simulink library "Room_Radiator"  (R2013b)
settings: Solver=ode45  StartTime=0.0  StopTime=10.0  RelTol=1e-3
libraries: carnot x17
settings Model: Creator=lena.frank  LastModifiedBy=drhf

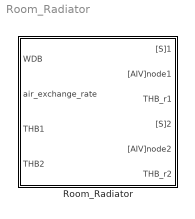
== system Room_Radiator ==
  Room_Radiator : Subsystem  mask(room){t0=20, temp_neighbour=20}
      mask prompts: t0 "start temperature of rooms in °C"; temp_neighbour "temperature of rooms above and below in °C"
      mask help:
      | The block models of a heat transfer characteristic of two neighbour rooms.
      | Use "look under mask" to set up the models parameters (initial conditions,
      | floors and wall characteristics...)
      mask init:
      | AIV_neighbour = [0 temp_neighbour temp_neighbour 0 0 0 0 0 0];
      | zonefloordist2grnd = 0;
      mask Help: web(fullfile(path_carnot('help'),'Room_Radiator.html'),'-helpbrowser')
      mask Display: plot(0,0,100,100,[30,30,60,60,30],[20,50,50,20,20],[47,47,56,56,47],[40,30,30,40,40],[42,42,34,34],[20,40,40,20],[62,45,28],[48,70,48])

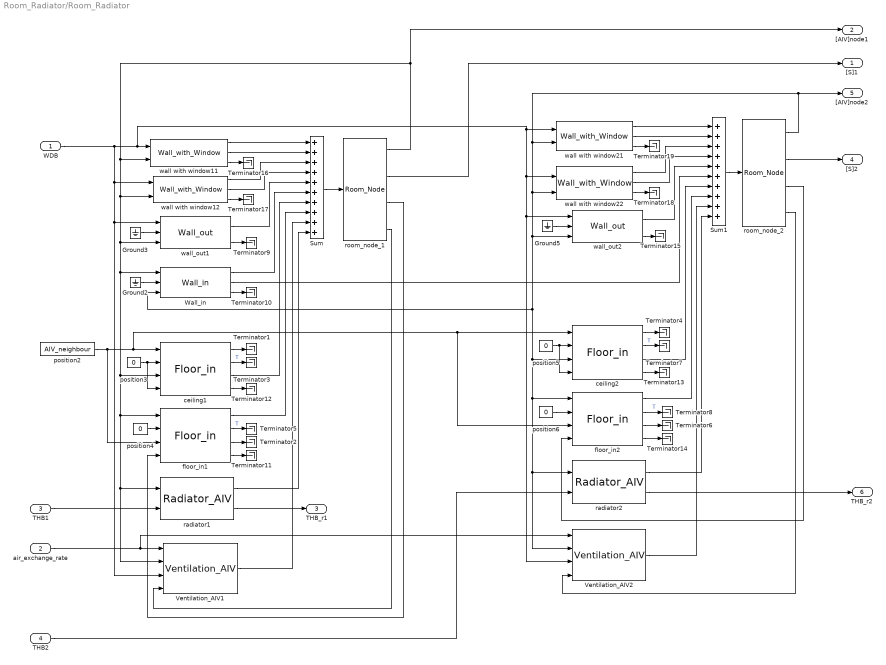
== system Room_Radiator/Room_Radiator ==
  WDB : Inport
  air_exchange_rate : Inport  Port=2
  THB1 : Inport  Port=3
  THB2 : Inport  Port=4
  Ground2 : Ground
  Ground3 : Ground
  Ground5 : Ground
  Sum : Sum  Inputs=10  SaturateOnIntegerOverflow=on  InputSameDT=on  OutDataTypeStr=Inherit: Same as first input
  Sum1 : Sum  Inputs=10  SaturateOnIntegerOverflow=on  InputSameDT=on  OutDataTypeStr=Inherit: Same as first input
  Terminator{1..19} (19 alike) : Terminator
  Ventilation_AIV1 : carnot/Source/Ventilation/Ventilation_AIV  co2=400
  Ventilation_AIV2 : carnot/Source/Ventilation/Ventilation_AIV  co2=400
  Wall_in : carnot/Load/Houses/wall_floor/Wall_in  wallsize=[2.5 5]  d=[0.015 0.38 0.02]  cond=[1.4 0.79 0.7]  cwall=[0.28 0.28 0.28]*3600  rho=[2000 1800 1400]  emission_in=0.96  dactive=-1  t0=20  tau=1000*3600
  ceiling1 : carnot/Load/Houses/wall_floor/Floor_in  wallsize=[5 5]  t0=20  d=[0.015 0.38 0.02]  cond=[1.4 0.79 0.7]  cwall=[0.28 0.28 0.28]*3600  rho=[2000 1800 1400]  misc=[.65 .65]  dactive=-1  tau=1000*3600
  ceiling2 : carnot/Load/Houses/wall_floor/Floor_in  wallsize=[5 5]  t0=20  d=[0.015 0.38 0.02]  cond=[1.4 0.79 0.7]  cwall=[0.28 0.28 0.28]*3600  rho=[2000 1800 1400]  misc=[.65 .65]  dactive=-1  tau=1000*3600
  floor_in1 : carnot/Load/Houses/wall_floor/Floor_in  wallsize=[5 5]  t0=20  d=[0.015 0.38 0.02]  cond=[1.4 0.79 0.7]  cwall=[0.28 0.28 0.28]*3600  rho=[2000 1800 1400]  misc=[.65 .65]  dactive=-1  tau=1000*3600
  floor_in2 : carnot/Load/Houses/wall_floor/Floor_in  wallsize=[5 5]  t0=20  d=[0.015 0.38 0.02]  cond=[1.4 0.79 0.7]  cwall=[0.28 0.28 0.28]*3600  rho=[2000 1800 1400]  misc=[.65 .65]  dactive=-1  tau=1000*3600
  position2 : Constant  Value=AIV_neighbour
  position{3..6} (4 alike) : Constant  Value=0
  radiator1 : carnot/Source/Heat_Exchanger/Radiator_AIV  pnom=500  dtnom=40  expo=1.3  mcap=5*4182  ra=0.47  tini=20  lin=0  qua=1000
  radiator2 : carnot/Source/Heat_Exchanger/Radiator_AIV  pnom=500  dtnom=40  expo=1.3  mcap=5*4182  ra=0.47  tini=20  lin=0  qua=1000
  room_node_1 : carnot/Load/Houses/room_nodes/Room_Node  zoneairvolume=5*5*2.5  zoneheight=2.5  zonestartTEMP=20  zonestartWATER=55  timeconst=100  heatperfect=natural  lookuptime=[0 24]*3600  lookupvalue=[20 20]  AirPressure=101300
  room_node_2 : carnot/Load/Houses/room_nodes/Room_Node  zoneairvolume=5*5*2.5  zoneheight=2.5  zonestartTEMP=20  zonestartWATER=55  timeconst=100  heatperfect=natural  lookuptime=[0 24]*3600  lookupvalue=[20 20]  AirPressure=101300
  wall with window11 : carnot/Load/Houses/wall_floor/Wall_with_Window  wallsize=[2.5 5]  windowsize=[1 2]  frame=0.1  pos=90  t0=20  tau=1000*3600  g=0.7
  wall with window12 : carnot/Load/Houses/wall_floor/Wall_with_Window  wallsize=[2.5 5]  windowsize=[1 2]  frame=0.1  pos=0  t0=20  tau=1000*3600  g=0.7
  wall with window21 : carnot/Load/Houses/wall_floor/Wall_with_Window  wallsize=[2.5 5]  windowsize=[1 2]  frame=0.1  pos=-90  t0=20  tau=1000*3600  g=0.7
  wall with window22 : carnot/Load/Houses/wall_floor/Wall_with_Window  wallsize=[2.5 5]  windowsize=[1 2]  frame=0.1  pos=0  t0=20  tau=1000*3600  g=0.7
  wall_out1 : carnot/Load/Houses/wall_floor/Wall_out  wallsize=[2.5 5]  pos=180  t0=20  d=[0.1 0.38]  cond=[0.04 0.79]  cwall=[0.28 0.28]*3600  rho=[900 1800]  reflectground=0.2  abs_emiss=[0.65 0.97 0.96]  tau=1000*3600  dactive=-1
  wall_out2 : carnot/Load/Houses/wall_floor/Wall_out  wallsize=[2.5 5]  pos=180  t0=20  d=[0.1 0.38]  cond=[0.04 0.79]  cwall=[0.28 0.28]*3600  rho=[900 1800]  reflectground=0.2  abs_emiss=[0.65 0.97 0.96]  tau=1000*3600  dactive=-1
  "[S]1" : Outport
  "[AIV]node1" : Outport  Port=2
  THB_r1 : Outport  Port=3
  "[S]2" : Outport  Port=4
  "[AIV]node2" : Outport  Port=5
  THB_r2 : Outport  Port=6
  wires:
  wall with window21/3 -> Terminator19/1
  wall with window22/3 -> Terminator18/1
  wall with window12/3 -> Terminator17/1
  wall with window11/3 -> Terminator16/1
  wall_out2/2 -> Terminator15/1
  floor_in2/4 -> Terminator14/1
  ceiling2/4 -> Terminator13/1
  ceiling1/4 -> Terminator12/1
  floor_in1/4 -> Terminator11/1
  Wall_in/3 -> Terminator10/1
  wall_out1/2 -> Terminator9/1
  Wall_in/1 -> Sum/6
  WDB/1 -> wall with window12/1, wall_out1/1, Ventilation_AIV1/3, wall with window11/1, wall with window21/1, wall with window22/1, wall_out2/1, Ventilation_AIV2/3
  wall with window11/1 -> Sum/1
  wall with window11/2 -> Sum/2
  wall with window12/1 -> Sum/3
  wall_out1/1 -> Sum/5
  wall with window12/2 -> Sum/4
  room_node_1/2 -> "[S]1"/1
  ceiling1/1 -> Terminator1/1
  ceiling1/2 -> Terminator3/1  "T"
  floor_in1/3 -> Terminator2/1
  position3/1 -> ceiling1/2, ceiling1/4
  floor_in1/1 -> Sum/8
  ceiling1/3 -> Sum/7
  Ventilation_AIV1/1 -> Sum/9
  THB1/1 -> radiator1/2
  radiator1/2 -> THB_r1/1
  room_node_1/4 -> Ventilation_AIV1/4
  room_node_1/3 -> floor_in1/4
  Ground2/1 -> Wall_in/2
  Ground3/1 -> wall_out1/2
  position2/1 -> floor_in1/3, ceiling1/1, floor_in2/3, ceiling2/1
  wall with window21/1 -> Sum1/1
  wall with window21/2 -> Sum1/2
  wall with window22/1 -> Sum1/3
  wall_out2/1 -> Sum1/5
  wall with window22/2 -> Sum1/4
  room_node_2/2 -> "[S]2"/1
  ceiling2/1 -> Terminator4/1
  ceiling2/2 -> Terminator7/1  "T"
  floor_in2/3 -> Terminator6/1
  position5/1 -> ceiling2/4, ceiling2/2
  floor_in2/1 -> Sum1/8
  ceiling2/3 -> Sum1/7
  Ventilation_AIV2/1 -> Sum1/9
  THB2/1 -> radiator2/2
  radiator2/2 -> THB_r2/1
  room_node_2/4 -> Ventilation_AIV2/4
  room_node_2/3 -> floor_in2/4
  Ground5/1 -> wall_out2/2
  Wall_in/2 -> Sum1/6
  air_exchange_rate/1 -> Ventilation_AIV1/1, Ventilation_AIV2/1
  room_node_1/1 -> wall with window11/2, wall with window12/2, wall_out1/3, Wall_in/1, ceiling1/3, floor_in1/1, radiator1/1, Ventilation_AIV1/2, "[AIV]node1"/1
  room_node_2/1 -> wall_out2/3, Wall_in/3, floor_in2/1, radiator2/1, Ventilation_AIV2/2, ceiling2/3, wall with window22/2, wall with window21/2, "[AIV]node2"/1
  floor_in2/2 -> Terminator8/1  "T"
  floor_in1/2 -> Terminator5/1  "T"
  position4/1 -> floor_in1/2
  position6/1 -> floor_in2/2
  radiator1/1 -> Sum/10
  radiator2/1 -> Sum1/10
  Sum/1 -> room_node_1/1
  Sum1/1 -> room_node_2/1
